simulink model "nonlinear_plant"  (Simulink 8.0)
settings: Solver=ode45  StartTime=0.0  StopTime=10  RelTol=1e-3
undefined symbols (not defined in the file): J, mgl
settings Model: Creator=dhoelzle  LastModifiedBy=dhoelzle

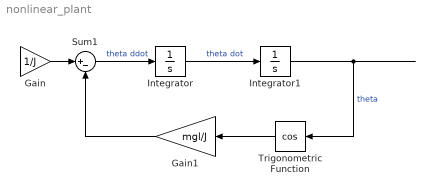
== system nonlinear_plant ==
  Gain : Gain  Gain=1/J
  Gain1 : Gain  Gain=mgl/J
  Integrator : Integrator
  Integrator1 : Integrator  InitialCondition=-.01
  Sum1 : Sum  Inputs=|+-
  Trigonometric Function : Trigonometry  Operator=cos
  wires:
  Sum1/1 -> Integrator/1  "theta ddot"
  Gain/1 -> Sum1/1
  Integrator/1 -> Integrator1/1  "theta dot"
  Integrator1/1 -> Trigonometric Function/1  "theta"
  Gain1/1 -> Sum1/2
  Trigonometric Function/1 -> Gain1/1
  ? -> Gain/1
